simulink model "to_point_minE"  (R2023b)
settings: Solver=FixedStepAuto  StartTime=0.0  StopTime=inf  RelTol=1e-3  EnableMultiTasking=on
model workspace (MAT data in the model file):
  G = 2001
undefined symbols (not defined in the file): c_t, f_max, f_min, Kd, Kp, M, W
libraries: rpi_blkst x3, robotcorelib x1
settings Model: SimulationMode=external  ExtModeTrigDuration=2  Creator=yabde  LastModifiedBy=yabde
settings SolverCC: PositivePriorityOrder=on
settings OptimizationCC: EnhancedBackFolding=on  PassReuseOutputArgsAs=Individual arguments  ZeroExternalMemoryAtStartup=off  ZeroInternalMemoryAtStartup=off  MaxStackSize=64  OptimizeBlockOrder=speed  DifferentSizesBufferReuse=on  OptimizationCustomize=off  EfficientTunableParamExpr=on
settings DebuggingCC: ParameterTunabilityLossMsg=error
settings HardwareCC: ProdBitPerLong=64  ProdLargestAtomicInteger=LongLong  ProdLargestAtomicFloat=Double  ProdLongLongMode=on  ProdHWDeviceType=ARM Compatible->ARM 64-bit (LP64)
settings RTWCC: Description=Embedded Coder  SystemTargetFile=ert.tlc  HardwareBoard=Raspberry Pi (64bit)  TemplateMakefile=ert_default_tmf  Toolchain=GNU GCC Embedded Linux  BuildConfiguration=Faster Runs
settings CodeAppCC: ForceParamTrailComments=on  IgnoreCustomStorageClasses=off  OperatorAnnotations=on  SimulinkDataObjDesc=on  SFDataObjDesc=on  InsertBlockDesc=on
settings ERTTargetCC: SupportVariableSizeSignals=on  ExtMode=on  ExtModeTransport=2  ExtModeStaticAlloc=on  ExtModeMaxTrigDuration=1000  ExtModeMexFile=ext_xcp  ExtModeMexArgs='192.168.0.31' 0 17725  ExtModeIntrfLevel=Level2 - Open

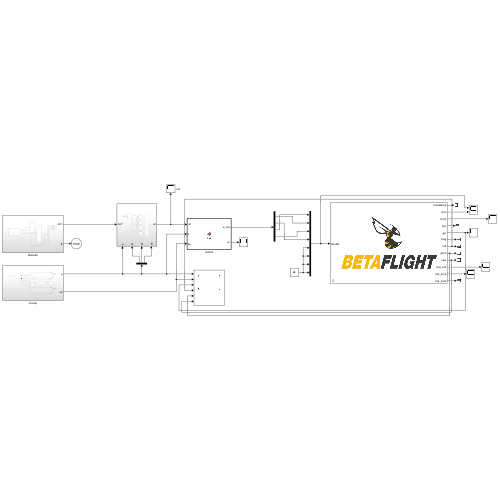
[thumbnail: Simulink's stored preview of the top-level diagram]
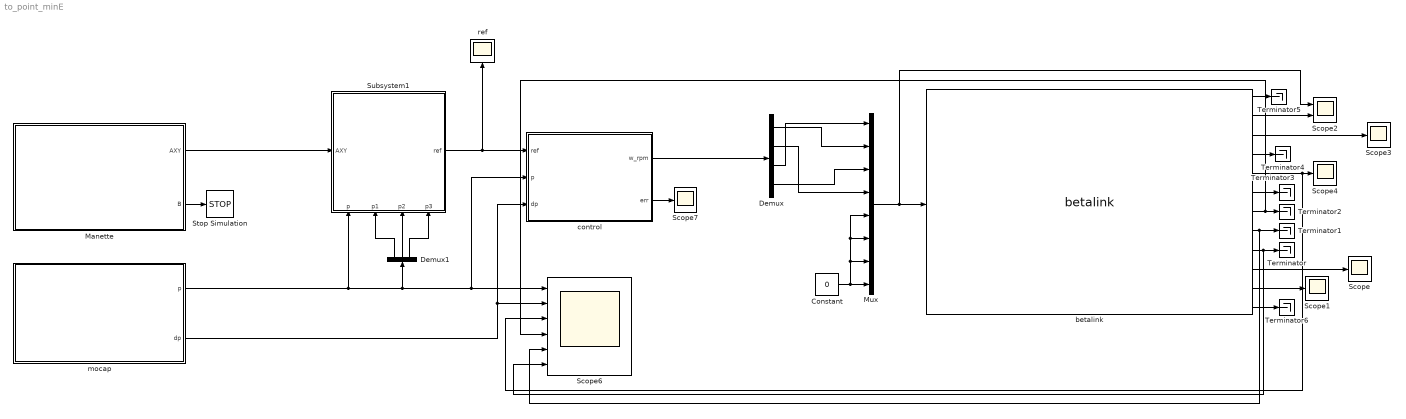
== system to_point_minE ==
  Constant : Constant  Value=0
  Demux : Demux
  Demux1 : Demux  Outputs=3
  Manette : Subsystem
  Mux : Mux  Inputs=8
  Scope{,1,3..4,7} (5 alike) : Scope
  Scope2 : Scope  NumInputPorts=2
  Scope6 : Scope  NumInputPorts=6
  Stop Simulation : Stop
  Subsystem1 : Subsystem
      settings: PortSchema="{\"entries\":[{\"content\":{\"sides\":[{\"content\":{\"connectorIds\":[\"In1\"]},\"type\":\"ConnectorPlacement.EquallySpacedRectSide\",\"uuid\":\"94773e7a-d08f-4fd8-82c5-ae10b9d7cfdf\"},{\"content\":{\"connectorIds\":[\"Out1\"],\"side\":\"RIGHT\"},\"type\":\"ConnectorPlacement.EquallySpacedRectSide\",\"uuid\":\"96dea559-8cff-42f7-9feb-e1d5469090e1\"},{\"content\":{\"side\":\"TOP\"},\"type\":\"ConnectorPlacement.EquallySpacedRectSide\",\"uuid\":\"bb642967-89fc-44ee-a1e7-4e0d63104ddc\"},{\"content\":{\"connectorIds\":[\"In2\",\"In3\",\"In4\",\"In5\"],\"side\":\"BOTTOM\"},\"type\":\"ConnectorPlacement.EquallySpacedRectSide\",\"uuid\":\"09ab3c6a-93c1-4021-b874-05a71fc68be9\"}]},\"type\":\"ConnectorPlacement.EquallySpacedConnector\",\"uuid\":\"47525873-1a41-4775-b5f8-ebd365059770\"}],\"packageUris\":[\"http://schema.mathworks.com/mf0/Connector/R2020b\"],\"version\":\"1.0\"}"
  Terminator{,1..6} (7 alike) : Terminator
  betalink : rpi_blkst/betalink  rpi_mask_usb_serial_number=1042260556  rpi_mask_Ts=0.01
      settings: SourceProductName=RPI Blockset
  control : MATLAB Function  TreatAsAtomicUnit=on
  mocap : Subsystem
  ref : Scope
  wires:
  Mux/1 -> betalink/1, Scope2/1
  Constant/1 -> Mux/5, Mux/6, Mux/7, Mux/8
  betalink/10 -> Scope/1
  betalink/11 -> Scope1/1
  betalink/2 -> Scope2/2
  betalink/3 -> Scope3/1
  betalink/5 -> Scope6/3, Scope4/1
  betalink/9 -> Scope6/6, Terminator/1
  betalink/8 -> Scope6/5, Terminator1/1
  betalink/7 -> Scope6/4, Terminator2/1
  betalink/6 -> Terminator3/1
  betalink/4 -> Terminator4/1
  betalink/12 -> Terminator6/1
  betalink/1 -> Terminator5/1
  mocap/2(dp) -> control/3(dp), Scope6/2
  control/1(w_rpm) -> Demux/1
  Demux/1 -> Mux/2
  Demux/2 -> Mux/4
  Demux/3 -> Mux/1
  Demux/4 -> Mux/3
  control/2(err) -> Scope7/1
  mocap/1(p) -> Demux1/1, control/2(p), Scope6/1, Subsystem1/2(p)
  Manette/2(B) -> Stop Simulation/1
  Subsystem1/1(ref) -> ref/1, control/1(ref)
  Manette/1(AXY) -> Subsystem1/1(AXY)
  Demux1/1 -> Subsystem1/3(p1)
  Demux1/2 -> Subsystem1/4(p2)
  Demux1/3 -> Subsystem1/5(p3)

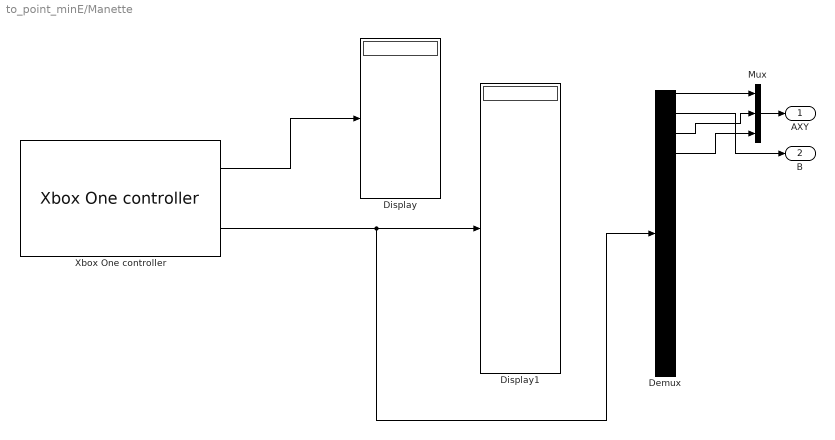
== system to_point_minE/Manette ==
  Demux : Demux  Outputs=15
  Display : Display
  Display1 : Display
  Mux : Mux  Inputs=3
  Xbox One controller : rpi_blkst/Xbox One controller  rpi_mask_ID=0  rpi_mask_Ts=0.01
      settings: SourceProductName=RPI Blockset
  AXY : Outport
  B : Outport  Port=2
  wires:
  Xbox One controller/1 -> Display/1
  Xbox One controller/2 -> Demux/1, Display1/1
  Demux/1 -> Mux/1
  Demux/4 -> Mux/3
  Mux/1 -> AXY/1
  Demux/2 -> B/1
  Demux/3 -> Mux/2

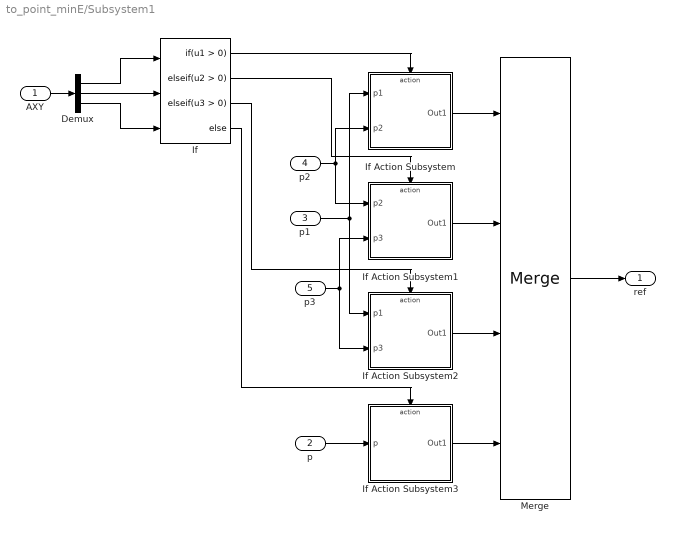
== system to_point_minE/Subsystem1 ==
  AXY : Inport
  p : Inport  Port=2
  p1 : Inport  Port=3
  p2 : Inport  Port=4
  p3 : Inport  Port=5
  Demux : Demux  Outputs=3
  If : If  NumInputs=3  ElseIfExpressions=u2 > 0, u3 > 0
  If Action Subsystem : Subsystem  TreatAsAtomicUnit=on
  If Action Subsystem1 : Subsystem  TreatAsAtomicUnit=on
  If Action Subsystem2 : Subsystem  TreatAsAtomicUnit=on
  If Action Subsystem3 : Subsystem  TreatAsAtomicUnit=on
  Merge : Merge  Inputs=4
  ref : Outport
  wires:
  p/1 -> If Action Subsystem3/1(p)
  If/1 -> If Action Subsystem/Action
  Demux/3 -> If/3
  p2/1 -> If Action Subsystem/2(p2), If Action Subsystem1/1(p2)
  p1/1 -> If Action Subsystem/1(p1), If Action Subsystem2/1(p1)
  If Action Subsystem/1(Out1) -> Merge/1
  If Action Subsystem1/1(Out1) -> Merge/2
  p3/1 -> If Action Subsystem1/2(p3), If Action Subsystem2/2(p3)
  If/3 -> If Action Subsystem2/Action
  If/4 -> If Action Subsystem3/Action
  If/2 -> If Action Subsystem1/Action
  If Action Subsystem2/1(Out1) -> Merge/3
  If Action Subsystem3/1(Out1) -> Merge/4
  Merge/1 -> ref/1
  Demux/2 -> If/2
  Demux/1 -> If/1
  AXY/1 -> Demux/1

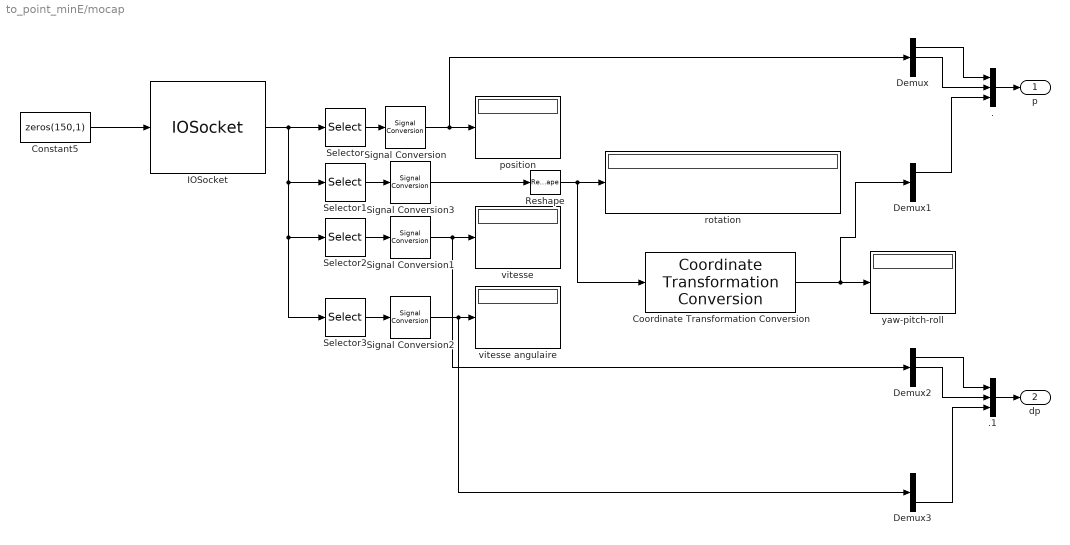
== system to_point_minE/mocap ==
  . : Mux  Inputs=3
  .1 : Mux  Inputs=3
  Constant5 : Constant  Value=zeros(150,1)
  Coordinate Transformation Conversion : robotcorelib/Coordinate Transformation Conversion  InputRepresentation=Rotation Matrix  InputEulerSequence=ZYX  ShowTrVecInputPort=on  OutputRepresentation=Euler Angles  OutputEulerSequence=ZYX  ShowTrVecOutputPort=on  SimulateUsing=Interpreted execution
  Demux{,1..3} (4 alike) : Demux  Outputs=3
  IOSocket : rpi_blkst/IOSocket  rpi_mask_Ts=0.01  rpi_mask_ip1=192  rpi_mask_ip2=168  rpi_mask_ip3=0  rpi_mask_ip4=13  rpi_mask_port=31415
      settings: SourceProductName=RPI Blockset
  Reshape : Reshape  OutputDimensionality=Customize  OutputDimensions=[3,3]
  Selector : Selector  IndexOptions=Index vector (dialog)  Indices=3:5  OutputSizes=1
  Selector1 : Selector  IndexOptions=Index vector (dialog)  Indices=6:14  OutputSizes=1
  Selector2 : Selector  IndexOptions=Index vector (dialog)  Indices=15:17  OutputSizes=1
  Selector3 : Selector  IndexOptions=Index vector (dialog)  Indices=18:20  OutputSizes=1
  Signal Conversion{,1..3} (4 alike) : SignalConversion  OverrideOpt=off
  position : Display
  rotation : Display
  vitesse : Display
  vitesse angulaire : Display
  yaw-pitch-roll : Display
  p : Outport
  dp : Outport  Port=2
  wires:
  Selector2/1 -> Signal Conversion1/1
  Signal Conversion1/1 -> Demux2/1, vitesse/1
  Signal Conversion2/1 -> Demux3/1, vitesse angulaire/1
  Selector/1 -> Signal Conversion/1
  Constant5/1 -> IOSocket/1
  Reshape/1 -> Coordinate Transformation Conversion/1, rotation/1
  IOSocket/1 -> Selector3/1, Selector2/1, Selector1/1, Selector/1
  Selector3/1 -> Signal Conversion2/1
  Signal Conversion/1 -> Demux/1, position/1
  Selector1/1 -> Signal Conversion3/1
  Signal Conversion3/1 -> Reshape/1
  Coordinate Transformation Conversion/1 -> Demux1/1, yaw-pitch-roll/1
  Demux/1 -> ./1
  Demux/2 -> ./2
  Demux1/1 -> ./3
  ./1 -> p/1
  .1/1 -> dp/1
  Demux2/2 -> .1/2
  Demux2/1 -> .1/1
  Demux3/3 -> .1/3

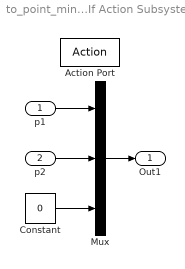
== system to_point_minE/Subsystem1/If Action Subsystem ==
  p1 : Inport
  p2 : Inport  Port=2
  Action Port : ActionPort  ActionPortLabel=if(u1 > 0)
  Constant : Constant  Value=0
  Mux : Mux  Inputs=3
  Out1 : Outport
  wires:
  p1/1 -> Mux/1
  p2/1 -> Mux/2
  Constant/1 -> Mux/3
  Mux/1 -> Out1/1

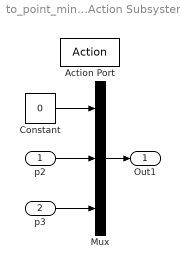
== system to_point_minE/Subsystem1/If Action Subsystem1 ==
  p2 : Inport
  p3 : Inport  Port=2
  Action Port : ActionPort  ActionPortLabel=elseif(u2 > 0)
  Constant : Constant  Value=0
  Mux : Mux  Inputs=3
  Out1 : Outport
  wires:
  Mux/1 -> Out1/1
  p3/1 -> Mux/3
  Constant/1 -> Mux/1
  p2/1 -> Mux/2

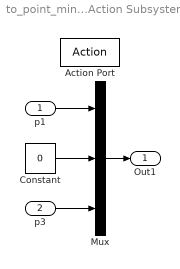
== system to_point_minE/Subsystem1/If Action Subsystem2 ==
  p1 : Inport
  p3 : Inport  Port=2
  Action Port : ActionPort  ActionPortLabel=elseif( u3 > 0)
  Constant : Constant  Value=0
  Mux : Mux  Inputs=3
  Out1 : Outport
  wires:
  p1/1 -> Mux/1
  Mux/1 -> Out1/1
  Constant/1 -> Mux/2
  p3/1 -> Mux/3

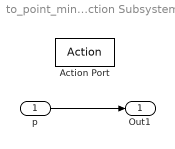
== system to_point_minE/Subsystem1/If Action Subsystem3 ==
  p : Inport
  Action Port : ActionPort  ActionPortLabel=else
  Out1 : Outport
  wires:
  p/1 -> Out1/1

== matlab function to_point_minE/control ==
  data: ref input; w_rpm output size=4; p input; dp input; Kp parameter; Kd parameter; M parameter; W parameter; c_t parameter; f_min parameter; f_max parameter; err output
function [w_rpm, err] = fcn(ref,p,dp,Kp,Kd,M,W,c_t,f_min,f_max)

thetaz = wrapToPi(p(3));
Rz = [cos(thetaz), -sin(thetaz), 0; 
      sin(thetaz),  cos(thetaz), 0;
      0,            0,           1];

W_rot = Rz * W;

% Effort désiré
err = ref - p;
err(3) = wrapToPi(err(3));
tau = M * (Kp * err);
% tau = M * (-Kd * dp + Kp * err);

% --- QP formulation : min ||W_rot*f - tau||^2 + lambda||f||^2 ---
lambda = 1e-3;  % petit régularisateur
H = 2*(W_rot'*W_rot + lambda*eye(4));
f_qp = -2*W_rot'*tau;
f0 = W \ tau;

% uniquement les bornes
options = optimoptions('quadprog','Display','off','Algorithm','active-set');
f = quadprog(H,f_qp,[],[],[],[],f_min,f_max,f0,options);

% Convertir en vitesses
w = sqrt(f ./ c_t);
w_rpm = w * 30/pi;

end
